simulink model "util_extra_hrn"  (R2014b)
settings: Solver=ode45  StartTime=0.0  StopTime=10.0  RelTol=1e-3
libraries: util_extra_lib x5, util_quat_lib x5
settings Model: Creator=ianmga  LastModifiedBy=mstewart
settings DataIOCC: SignalLoggingSaveFormat=ModelDataLogs
settings OptimizationCC: ExpressionDepthLimit=2147483647
settings DebuggingCC: UnderspecifiedInitializationDetection=Classic  MergeDetectMultiDrivingBlocksExec=none  FcnCallInpInsideContextMsg=UseLocalSettings  StateNameClashWarn=warning
settings GRTTargetCC: CombineOutputUpdateFcns=off  GRTInterface=on

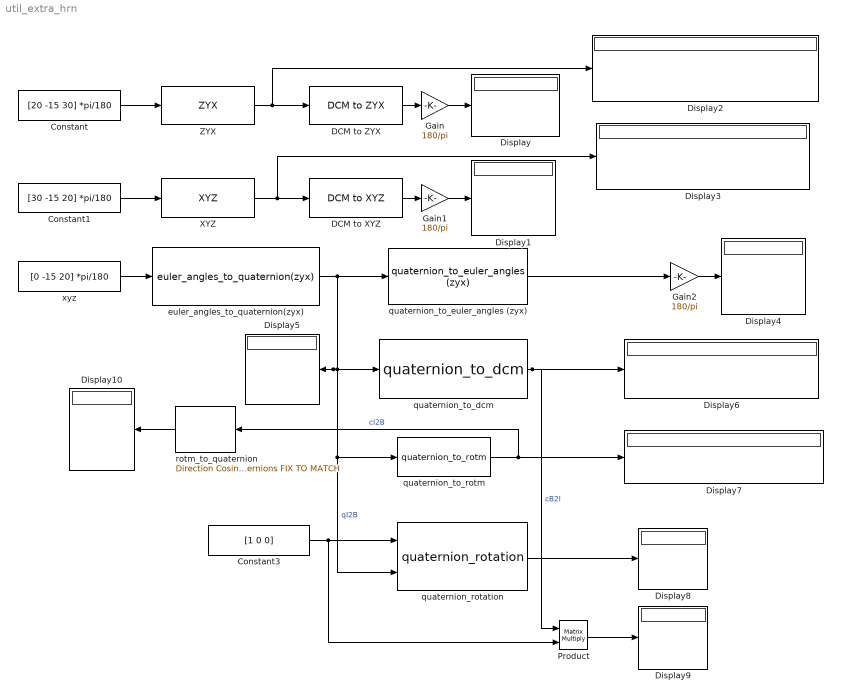
== system util_extra_hrn ==
  Constant : Constant  Value=[20 -15 30] *pi/180
  Constant1 : Constant  Value=[30 -15 20] *pi/180
  Constant3 : Constant  Value=[1 0 0]
  DCM to XYZ : util_extra_lib/DCM to XYZ
  DCM to ZYX : util_extra_lib/DCM to ZYX
  Display{,1..10} (11 alike) : Display
  Gain : Gain  Gain=180/pi
  Gain1 : Gain  Gain=180/pi
  Gain2 : Gain  Gain=180/pi
  Product : Product  Multiplication=Matrix(*)  RndMeth=Zero
  XYZ : util_extra_lib/XYZ
  ZYX : util_extra_lib/ZYX
  euler_angles_to_quaternion(zyx) : util_quat_lib/euler_angles_to_quaternion(zyx)  SystemSampleTime=-1
  quaternion_rotation : util_quat_lib/quaternion_rotation  SystemSampleTime=-1
  quaternion_to_dcm : util_quat_lib/quaternion_to_dcm  SystemSampleTime=-1
  quaternion_to_euler_angles (zyx) : util_quat_lib/quaternion_to_euler_angles (zyx)  SystemSampleTime=-1
  quaternion_to_rotm : util_quat_lib/quaternion_to_rotm  SystemSampleTime=-1
  rotm_to_quaternion : util_extra_lib/Direction Cosine Matrix  to Quaternions FIX TO MATCH  SystemSampleTime=-1
  xyz : Constant  Value=[0 -15 20] *pi/180
  wires:
  Constant/1 -> ZYX/1
  Constant1/1 -> XYZ/1
  XYZ/1 -> DCM to XYZ/1, Display3/1
  ZYX/1 -> DCM to ZYX/1, Display2/1
  DCM to ZYX/1 -> Gain/1
  DCM to XYZ/1 -> Gain1/1
  Gain/1 -> Display/1
  Gain1/1 -> Display1/1
  euler_angles_to_quaternion(zyx)/1 -> quaternion_to_euler_angles (zyx)/1, Display5/1, quaternion_to_dcm/1, quaternion_to_rotm/1, quaternion_rotation/2  "qI2B"
  Gain2/1 -> Display4/1
  quaternion_to_euler_angles (zyx)/1 -> Gain2/1
  quaternion_to_rotm/1 -> Display7/1, rotm_to_quaternion/1  "cI2B"
  quaternion_to_dcm/1 -> Display6/1, Product/1  "cB2I"
  xyz/1 -> euler_angles_to_quaternion(zyx)/1
  Constant3/1 -> quaternion_rotation/1, Product/2
  quaternion_rotation/1 -> Display8/1
  Product/1 -> Display9/1
  rotm_to_quaternion/1 -> Display10/1
